simulink model "DigitalModulation_ASK"  (R2023b)
settings: Solver=VariableStepAuto  StartTime=0.0  StopTime=10.0  RelTol=1e-3
settings Model: Creator=Aman Tripathi  LastModifiedBy=Spedrik Webster

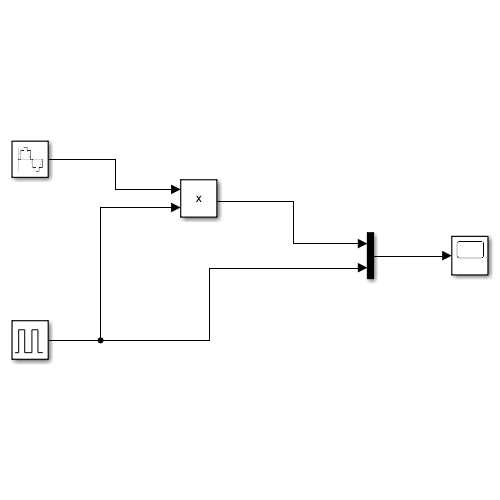
[thumbnail: Simulink's stored preview of the top-level diagram]
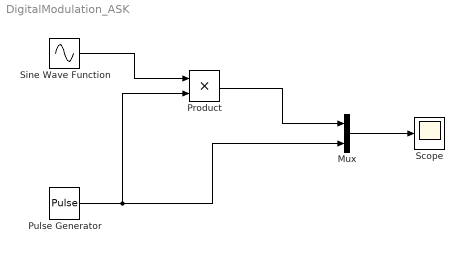
== system DigitalModulation_ASK ==
  Mux : Mux  Inputs=2
  Product : Product
  Pulse Generator : DiscretePulseGenerator  PulseType=Time based  PulseWidth=50
  Scope : Scope
  Sine Wave Function : Sin  Frequency=50  SampleTime=1/5000
  wires:
  Sine Wave Function/1 -> Product/1
  Pulse Generator/1 -> Product/2, Mux/2
  Product/1 -> Mux/1
  Mux/1 -> Scope/1
